simulink library "PC_Simulator_Lib"  (Simulink 8.2)
settings: Solver=ode45  StartTime=0.0  StopTime=10.0  RelTol=1e-3
values from neighbouring files (symbols this model uses):
  data = [r1 r2 r3 r4 L1 L2 L3 L4]    [strasse_Bedatung_HNI_ITI.m]
  distSameLane = 60    [InitialisationsEnv.m]
  eng_speed = [0 60 120 180 240 300 360 420 480 540 600 660 ... (101 elements, 1x101)]    [engine_table.mat]    (also in motor_parameter_calc.m = omega)
  Heading_init = 0    [Start.m]
  inertiaLateral = 25*(radiusWheel)^2    (= 4.129024)    [Start.m]
  laneWidth = 3.6    [InitialisationsEnv.m]    (also in strasse_Bedatung_HNI_ITI.m)
  omega_engine = [0.000000 150.000000 500.000000 1000.000000 1500.000000 2000.000000 2500.000000 3000.000000 3500.000000 4000.000000 4500.000000 5000.000000 5500.000000 6000.000000]    [friction_tables.m]
  omega_max = 6000    [engine_table.mat]    (also in motor_parameter_calc.m)
  omega_wheel = [0 20 40 60 80 100 122 143.7 164]    [friction_tables.m]
  para_Fellow_8_Points = ADAS.Fellow_8_Points    [ADAS_parameters.m]
  position_start_x = [x1 x2 x3 x4 x5 x6 x7]    [strasse_Bedatung_HNI_ITI.m]
  position_start_y = [y1 y2 y3 y4 y5 y6 y7]    [strasse_Bedatung_HNI_ITI.m]
  rad3rdLine = 57.2    [InitialisationsEnv.m]    (also in strasse_Bedatung_HNI_ITI.m)
  radiusWheel = 16*2.54/100    (= 0.4064)    [Start.m]
  s_values = [S1 S2 S3 S4 S5 S6 S7]    [strasse_Bedatung_HNI_ITI.m]
  segmentLimits = [segment1EndThirdLine                   segment2EndThirdLine                   segment3EndThirdLine                   segment4EndThirdLine                   segment5EndThirdLine                   segment6EndThirdLine                   segment7EndThirdLine                   segment8EndThirdLine                   ]    [InitialisationsEnv.m]    (also in strasse_Bedatung_HNI_ITI.m)
  setPosT = [-1.8 -5.4 -1.8 -5.4 -1.8 -5.4 -1.8 -5.4 -1.8 -5.4]    [InitialisationsEnv.m]
  torque = [297.089227105 300.997600937 304.800343044 308.497453426 312.088932082 315.574779014 318.95499422 322.229577701 325.398529457 328.461849487 331.419537793 334.271594373 ... (101 elements, 1x101)]    [engine_table.mat]    (also in motor_parameter_calc.m = g)
  Torque_lost = [0.000000 -8.777780 -15.000000 -26.800000 -29.600000 -32.700000 -35.900000 -39.300000 -42.800000 -46.500000 -50.300000 -54.300000 -58.500000 -62.800000 ]*0.6    [friction_tables.m]
  Torque_lost_wheel = [0.8 0.8 0.75 0.7 0.4 0.3 0.2 0.07 0.07]*0.2    [friction_tables.m]
  X_init = 0    [Start.m]
  Y_init = 1.8    [Start.m]
  Z_init = 0    [Start.m]
undefined symbols (not defined in the file or in its folder): Acc_Pedal, ADAS, Brake_Pedal, Joystick, Newton, Para, Raphson, Standard_Devices, Steering_Wheel_Angle, UDP_Protocol
libraries: simulink x43, rtwinlib x7, dspnetwork x2, simulink_extras x1, vrlib x1
(part 3 of 13)

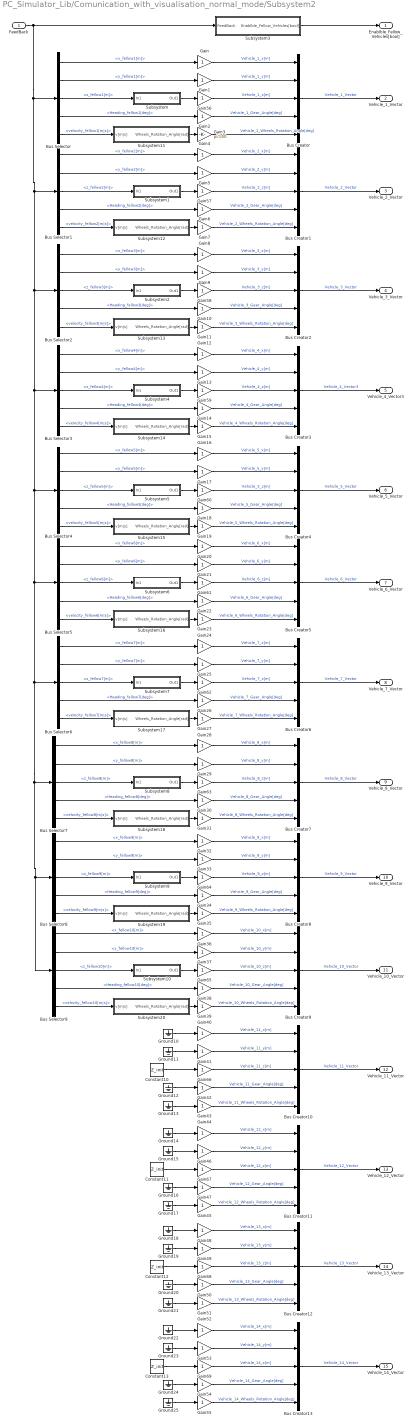
== system PC_Simulator_Lib/Comunication_with_visualisation_normal_mode/Subsystem2 ==
  FeedBack : Inport
  Bus Creator{,1..13} (14 alike) : BusCreator  Inputs=5
  Bus Selector : BusSelector  OutputSignals=Environment.fellow_car_1.x_fellow1[m],Environment.fellow_car_1.y_fellow1[m],Environment.fellow_car_1.z_fellow1[m],Environment.fellow_car_1.Heading_fellow1[deg],Environment.fellow_car_1.velocity_fellow1[m|s]
  Bus Selector1 : BusSelector  OutputSignals=Environment.fellow_car_2.x_fellow2[m],Environment.fellow_car_2.y_fellow2[m],Environment.fellow_car_2.z_fellow2[m],Environment.fellow_car_2.Heading_fellow2[deg],Environment.fellow_car_2.velocity_fellow2[m|s]
  Bus Selector2 : BusSelector  OutputSignals=Environment.fellow_car_3.x_fellow3[m],Environment.fellow_car_3.y_fellow3[m],Environment.fellow_car_3.z_fellow3[m],Environment.fellow_car_3.Heading_fellow3[deg],Environment.fellow_car_3.velocity_fellow3[m|s]
  Bus Selector3 : BusSelector  OutputSignals=Environment.fellow_car_4.x_fellow4[m],Environment.fellow_car_4.y_fellow4[m],Environment.fellow_car_4.z_fellow4[m],Environment.fellow_car_4.Heading_fellow4[deg],Environment.fellow_car_4.velocity_fellow4[m|s]
  Bus Selector4 : BusSelector  OutputSignals=Environment.fellow_car_5.x_fellow5[m],Environment.fellow_car_5.y_fellow5[m],Environment.fellow_car_5.z_fellow5[m],Environment.fellow_car_5.Heading_fellow5[deg],Environment.fellow_car_5.velocity_fellow5[m|s]
  Bus Selector5 : BusSelector  OutputSignals=Environment.fellow_car_6.x_fellow6[m],Environment.fellow_car_6.y_fellow6[m],Environment.fellow_car_6.z_fellow6[m],Environment.fellow_car_6.Heading_fellow6[deg],Environment.fellow_car_6.velocity_fellow6[m|s]
  Bus Selector6 : BusSelector  OutputSignals=Environment.fellow_car_7.x_fellow7[m],Environment.fellow_car_7.y_fellow7[m],Environment.fellow_car_7.z_fellow7[m],Environment.fellow_car_7.Heading_fellow7[deg],Environment.fellow_car_7.velocity_fellow7[m|s]
  Bus Selector7 : BusSelector  OutputSignals=Environment.fellow_car_8.x_fellow8[m],Environment.fellow_car_8.y_fellow8[m],Environment.fellow_car_8.z_fellow8[m],Environment.fellow_car_8.Heading_fellow8[deg],Environment.fellow_car_8.velocity_fellow8[m|s]
  Bus Selector8 : BusSelector  OutputSignals=Environment.fellow_car_9.x_fellow9[m],Environment.fellow_car_9.y_fellow9[m],Environment.fellow_car_9.z_fellow9[m],Environment.fellow_car_9.Heading_fellow9[deg],Environment.fellow_car_9.velocity_fellow9[m|s]
  Bus Selector9 : BusSelector  OutputSignals=Environment.fellow_car_10.x_fellow10[m],Environment.fellow_car_10.y_fellow10[m],Environment.fellow_car_10.z_fellow10[m],Environment.fellow_car_10.Heading_fellow10[deg],Environment.fellow_car_10.velocity_fellow10[m|s]
  Constant{10..13} (4 alike) : Constant  Value=Z_init
  Gain{,1..2,4..69} (69 alike) : Gain
  Gain3 : Gain  Gain=pi/180
  Ground{10..25} (16 alike) : Ground
  Subsystem : Subsystem
  Subsystem1 : Subsystem
  Subsystem10 : Subsystem
  Subsystem11 : Subsystem
  Subsystem12 : Subsystem
  Subsystem13 : Subsystem
  Subsystem14 : Subsystem
  Subsystem15 : Subsystem
  Subsystem16 : Subsystem
  Subsystem17 : Subsystem
  Subsystem18 : Subsystem
  Subsystem19 : Subsystem
  Subsystem2 : Subsystem
  Subsystem20 : Subsystem
  Subsystem3 : Subsystem
  Subsystem4 : Subsystem
  Subsystem5 : Subsystem
  Subsystem6 : Subsystem
  Subsystem7 : Subsystem
  Subsystem8 : Subsystem
  Subsystem9 : Subsystem
  Enablble_Fellow_Vehicles[bool] : Outport
  Vehicle_1_Vector : Outport  Port=2
  Vehicle_2_Vector : Outport  Port=3
  Vehicle_3_Vector : Outport  Port=4
  Vehicle_4_Vector3 : Outport  Port=5
  Vehicle_5_Vector : Outport  Port=6
  Vehicle_6_Vector : Outport  Port=7
  Vehicle_7_Vector : Outport  Port=8
  Vehicle_8_Vector : Outport  Port=9
  Vehicle_9_Vector : Outport  Port=10
  Vehicle_10_Vector : Outport  Port=11
  Vehicle_11_Vector : Outport  Port=12
  Vehicle_12_Vector : Outport  Port=13
  Vehicle_13_Vector : Outport  Port=14
  Vehicle_14_Vector : Outport  Port=15
  wires:
  Bus Creator/1 -> Vehicle_1_Vector/1  "Vehicle_1_Vector"
  Bus Creator1/1 -> Vehicle_2_Vector/1  "Vehicle_2_Vector"
  Bus Creator2/1 -> Vehicle_3_Vector/1  "Vehicle_3_Vector"
  Bus Creator3/1 -> Vehicle_4_Vector3/1  "Vehicle_4_Vector3"
  Bus Creator4/1 -> Vehicle_5_Vector/1  "Vehicle_5_Vector"
  Bus Creator5/1 -> Vehicle_6_Vector/1  "Vehicle_6_Vector"
  Bus Creator6/1 -> Vehicle_7_Vector/1  "Vehicle_7_Vector"
  Bus Creator7/1 -> Vehicle_8_Vector/1  "Vehicle_8_Vector"
  Bus Creator8/1 -> Vehicle_9_Vector/1  "Vehicle_9_Vector"
  Bus Creator9/1 -> Vehicle_10_Vector/1  "Vehicle_10_Vector"
  Bus Creator10/1 -> Vehicle_11_Vector/1  "Vehicle_11_Vector"
  Bus Creator11/1 -> Vehicle_12_Vector/1  "Vehicle_12_Vector"
  Bus Creator12/1 -> Vehicle_13_Vector/1  "Vehicle_13_Vector"
  Bus Creator13/1 -> Vehicle_14_Vector/1  "Vehicle_14_Vector"
  Gain/1 -> Bus Creator/1  "Vehicle_1_x[m]"
  Gain1/1 -> Bus Creator/2  "Vehicle_1_y[m]"
  Gain56/1 -> Bus Creator/3  "Vehicle_1_z[m]"
  Gain2/1 -> Bus Creator/4  "Vehicle_1_Gear_Angle[deg]"
  Gain3/1 -> Bus Creator/5  "Vehicle_1_Wheels_Rotation_Angle[deg]"
  Gain4/1 -> Bus Creator1/1  "Vehicle_2_x[m]"
  Gain5/1 -> Bus Creator1/2  "Vehicle_2_y[m]"
  Gain57/1 -> Bus Creator1/3  "Vehicle_2_z[m]"
  Gain6/1 -> Bus Creator1/4  "Vehicle_2_Gear_Angle[deg]"
  Gain7/1 -> Bus Creator1/5  "Vehicle_2_Wheels_Rotation_Angle[deg]"
  Gain8/1 -> Bus Creator2/1  "Vehicle_3_x[m]"
  Gain9/1 -> Bus Creator2/2  "Vehicle_3_y[m]"
  Gain58/1 -> Bus Creator2/3  "Vehicle_3_z[m]"
  Gain10/1 -> Bus Creator2/4  "Vehicle_3_Gear_Angle[deg]"
  Gain11/1 -> Bus Creator2/5  "Vehicle_3_Wheels_Rotation_Angle[deg]"
  Gain12/1 -> Bus Creator3/1  "Vehicle_4_x[m]"
  Gain13/1 -> Bus Creator3/2  "Vehicle_4_y[m]"
  Gain59/1 -> Bus Creator3/3  "Vehicle_4_z[m]"
  Gain14/1 -> Bus Creator3/4  "Vehicle_4_Gear_Angle[deg]"
  Gain15/1 -> Bus Creator3/5  "Vehicle_4_Wheels_Rotation_Angle[deg]"
  Gain16/1 -> Bus Creator4/1  "Vehicle_5_x[m]"
  Gain17/1 -> Bus Creator4/2  "Vehicle_5_y[m]"
  Gain60/1 -> Bus Creator4/3  "Vehicle_5_z[m]"
  Gain18/1 -> Bus Creator4/4  "Vehicle_5_Gear_Angle[deg]"
  Gain19/1 -> Bus Creator4/5  "Vehicle_5_Wheels_Rotation_Angle[deg]"
  Gain20/1 -> Bus Creator5/1  "Vehicle_6_x[m]"
  Gain21/1 -> Bus Creator5/2  "Vehicle_6_y[m]"
  Gain61/1 -> Bus Creator5/3  "Vehicle_6_z[m]"
  Gain22/1 -> Bus Creator5/4  "Vehicle_6_Gear_Angle[deg]"
  Gain23/1 -> Bus Creator5/5  "Vehicle_6_Wheels_Rotation_Angle[deg]"
  Gain24/1 -> Bus Creator6/1  "Vehicle_7_x[m]"
  Gain25/1 -> Bus Creator6/2  "Vehicle_7_y[m]"
  Gain62/1 -> Bus Creator6/3  "Vehicle_7_z[m]"
  Gain26/1 -> Bus Creator6/4  "Vehicle_7_Gear_Angle[deg]"
  Gain27/1 -> Bus Creator6/5  "Vehicle_7_Wheels_Rotation_Angle[deg]"
  Gain28/1 -> Bus Creator7/1  "Vehicle_8_x[m]"
  Gain29/1 -> Bus Creator7/2  "Vehicle_8_y[m]"
  Gain63/1 -> Bus Creator7/3  "Vehicle_8_z[m]"
  Gain30/1 -> Bus Creator7/4  "Vehicle_8_Gear_Angle[deg]"
  Gain31/1 -> Bus Creator7/5  "Vehicle_8_Wheels_Rotation_Angle[deg]"
  Gain32/1 -> Bus Creator8/1  "Vehicle_9_x[m]"
  Gain33/1 -> Bus Creator8/2  "Vehicle_9_y[m]"
  Gain64/1 -> Bus Creator8/3  "Vehicle_9_z[m]"
  Gain34/1 -> Bus Creator8/4  "Vehicle_9_Gear_Angle[deg]"
  Gain35/1 -> Bus Creator8/5  "Vehicle_9_Wheels_Rotation_Angle[deg]"
  Gain36/1 -> Bus Creator9/1  "Vehicle_10_x[m]"
  Gain37/1 -> Bus Creator9/2  "Vehicle_10_y[m]"
  Gain65/1 -> Bus Creator9/3  "Vehicle_10_z[m]"
  Gain38/1 -> Bus Creator9/4  "Vehicle_10_Gear_Angle[deg]"
  Gain39/1 -> Bus Creator9/5  "Vehicle_10_Wheels_Rotation_Angle[deg]"
  Gain40/1 -> Bus Creator10/1  "Vehicle_11_x[m]"
  Gain41/1 -> Bus Creator10/2  "Vehicle_11_y[m]"
  Gain66/1 -> Bus Creator10/3  "Vehicle_11_z[m]"
  Gain42/1 -> Bus Creator10/4  "Vehicle_11_Gear_Angle[deg]"
  Gain43/1 -> Bus Creator10/5  "Vehicle_11_Wheels_Rotation_Angle[deg]"
  Gain44/1 -> Bus Creator11/1  "Vehicle_12_x[m]"
  Gain46/1 -> Bus Creator11/2  "Vehicle_12_y[m]"
  Gain67/1 -> Bus Creator11/3  "Vehicle_12_z[m]"
  Gain47/1 -> Bus Creator11/4  "Vehicle_12_Gear_Angle[deg]"
  Gain45/1 -> Bus Creator11/5  "Vehicle_12_Wheels_Rotation_Angle[deg]"
  Gain48/1 -> Bus Creator12/1  "Vehicle_13_x[m]"
  Gain49/1 -> Bus Creator12/2  "Vehicle_13_y[m]"
  Gain68/1 -> Bus Creator12/3  "Vehicle_13_z[m]"
  Gain50/1 -> Bus Creator12/4  "Vehicle_13_Gear_Angle[deg]"
  Gain51/1 -> Bus Creator12/5  "Vehicle_13_Wheels_Rotation_Angle[deg]"
  Gain52/1 -> Bus Creator13/1  "Vehicle_14_x[m]"
  Gain53/1 -> Bus Creator13/2  "Vehicle_14_y[m]"
  Gain69/1 -> Bus Creator13/3  "Vehicle_14_z[m]"
  Gain54/1 -> Bus Creator13/4  "Vehicle_14_Gear_Angle[deg]"
  Gain55/1 -> Bus Creator13/5  "Vehicle_14_Wheels_Rotation_Angle[deg]"
  Subsystem3/1(Enablble_Fellow_Vehicles[bool]) -> Enablble_Fellow_Vehicles[bool]/1
  Subsystem5/1(Out1) -> Gain60/1
  Subsystem6/1(Out1) -> Gain61/1
  Subsystem7/1(Out1) -> Gain62/1
  Subsystem8/1(Out1) -> Gain63/1
  Subsystem9/1(Out1) -> Gain64/1
  Subsystem10/1(Out1) -> Gain65/1
  Constant10/1 -> Gain66/1
  Constant11/1 -> Gain67/1
  Constant12/1 -> Gain68/1
  Constant13/1 -> Gain69/1
  Subsystem/1(Out1) -> Gain56/1
  Bus Selector/1 -> Gain/1  "<x_fellow1[m]>"
  Bus Selector/2 -> Gain1/1  "<y_fellow1[m]>"
  Bus Selector/3 -> Subsystem/1(In1)  "<z_fellow1[m]>"
  Bus Selector/4 -> Gain2/1  "<Heading_fellow1[deg]>"
  Ground10/1 -> Gain40/1
  Ground11/1 -> Gain41/1
  Ground12/1 -> Gain42/1
  Ground13/1 -> Gain43/1
  Ground14/1 -> Gain44/1
  Ground15/1 -> Gain46/1
  Ground16/1 -> Gain47/1
  Ground17/1 -> Gain45/1
  Ground18/1 -> Gain48/1
  Ground19/1 -> Gain49/1
  Ground20/1 -> Gain50/1
  Ground21/1 -> Gain51/1
  Ground22/1 -> Gain52/1
  Ground23/1 -> Gain53/1
  Ground24/1 -> Gain54/1
  Ground25/1 -> Gain55/1
  Subsystem1/1(Out1) -> Gain57/1
  Subsystem2/1(Out1) -> Gain58/1
  Subsystem4/1(Out1) -> Gain59/1
  FeedBack/1 -> Bus Selector9/1, Bus Selector8/1, Bus Selector7/1, Bus Selector6/1, Bus Selector5/1, Bus Selector4/1, Bus Selector3/1, Bus Selector2/1, Bus Selector1/1, Bus Selector/1, Subsystem3/1(FeedBack)
  Bus Selector1/3 -> Subsystem1/1(In1)  "<z_fellow2[m]>"
  Bus Selector1/1 -> Gain4/1  "<x_fellow2[m]>"
  Bus Selector1/2 -> Gain5/1  "<y_fellow2[m]>"
  Bus Selector1/4 -> Gain6/1  "<Heading_fellow2[deg]>"
  Bus Selector2/3 -> Subsystem2/1(In1)  "<z_fellow3[m]>"
  Bus Selector2/1 -> Gain8/1  "<x_fellow3[m]>"
  Bus Selector2/2 -> Gain9/1  "<y_fellow3[m]>"
  Bus Selector2/4 -> Gain10/1  "<Heading_fellow3[deg]>"
  Bus Selector3/3 -> Subsystem4/1(In1)  "<z_fellow4[m]>"
  Bus Selector3/1 -> Gain12/1  "<x_fellow4[m]>"
  Bus Selector3/2 -> Gain13/1  "<y_fellow4[m]>"
  Bus Selector3/4 -> Gain14/1  "<Heading_fellow4[deg]>"
  Bus Selector4/3 -> Subsystem5/1(In1)  "<z_fellow5[m]>"
  Bus Selector4/1 -> Gain16/1  "<x_fellow5[m]>"
  Bus Selector4/2 -> Gain17/1  "<y_fellow5[m]>"
  Bus Selector4/4 -> Gain18/1  "<Heading_fellow5[deg]>"
  Bus Selector5/3 -> Subsystem6/1(In1)  "<z_fellow6[m]>"
  Bus Selector5/1 -> Gain20/1  "<x_fellow6[m]>"
  Bus Selector5/2 -> Gain21/1  "<y_fellow6[m]>"
  Bus Selector5/4 -> Gain22/1  "<Heading_fellow6[deg]>"
  Bus Selector6/3 -> Subsystem7/1(In1)  "<z_fellow7[m]>"
  Bus Selector6/1 -> Gain24/1  "<x_fellow7[m]>"
  Bus Selector6/2 -> Gain25/1  "<y_fellow7[m]>"
  Bus Selector6/4 -> Gain26/1  "<Heading_fellow7[deg]>"
  Bus Selector7/3 -> Subsystem8/1(In1)  "<z_fellow8[m]>"
  Bus Selector7/1 -> Gain28/1  "<x_fellow8[m]>"
  Bus Selector7/2 -> Gain29/1  "<y_fellow8[m]>"
  Bus Selector7/4 -> Gain30/1  "<Heading_fellow8[deg]>"
  Bus Selector8/3 -> Subsystem9/1(In1)  "<z_fellow9[m]>"
  Bus Selector8/1 -> Gain32/1  "<x_fellow9[m]>"
  Bus Selector8/2 -> Gain33/1  "<y_fellow9[m]>"
  Bus Selector8/4 -> Gain34/1  "<Heading_fellow9[deg]>"
  Bus Selector9/3 -> Subsystem10/1(In1)  "<z_fellow10[m]>"
  Bus Selector9/1 -> Gain36/1  "<x_fellow10[m]>"
  Bus Selector9/2 -> Gain37/1  "<y_fellow10[m]>"
  Bus Selector9/4 -> Gain38/1  "<Heading_fellow10[deg]>"
  Subsystem11/1(Wheels_Rotation_Angle[rad]) -> Gain3/1
  Subsystem12/1(Wheels_Rotation_Angle[rad]) -> Gain7/1
  Subsystem13/1(Wheels_Rotation_Angle[rad]) -> Gain11/1
  Subsystem14/1(Wheels_Rotation_Angle[rad]) -> Gain15/1
  Subsystem15/1(Wheels_Rotation_Angle[rad]) -> Gain19/1
  Subsystem16/1(Wheels_Rotation_Angle[rad]) -> Gain23/1
  Subsystem17/1(Wheels_Rotation_Angle[rad]) -> Gain27/1
  Subsystem18/1(Wheels_Rotation_Angle[rad]) -> Gain31/1
  Subsystem19/1(Wheels_Rotation_Angle[rad]) -> Gain35/1
  Subsystem20/1(Wheels_Rotation_Angle[rad]) -> Gain39/1
  Bus Selector/5 -> Subsystem11/1(v[m|s])  "<velocity_fellow1[m|s]>"
  Bus Selector1/5 -> Subsystem12/1(v[m|s])  "<velocity_fellow2[m|s]>"
  Bus Selector9/5 -> Subsystem20/1(v[m|s])  "<velocity_fellow10[m|s]>"
  Bus Selector8/5 -> Subsystem19/1(v[m|s])  "<velocity_fellow9[m|s]>"
  Bus Selector7/5 -> Subsystem18/1(v[m|s])  "<velocity_fellow8[m|s]>"
  Bus Selector6/5 -> Subsystem17/1(v[m|s])  "<velocity_fellow7[m|s]>"
  Bus Selector5/5 -> Subsystem16/1(v[m|s])  "<velocity_fellow6[m|s]>"
  Bus Selector4/5 -> Subsystem15/1(v[m|s])  "<velocity_fellow5[m|s]>"
  Bus Selector3/5 -> Subsystem14/1(v[m|s])  "<velocity_fellow4[m|s]>"
  Bus Selector2/5 -> Subsystem13/1(v[m|s])  "<velocity_fellow3[m|s]>"

== system PC_Simulator_Lib/Comunication_with_visualisation_normal_mode/Subsystem3 ==
  In1 : Inport
  Add : Sum
  Constant : Constant  Value=1000
  Gain1 : Gain  Gain=60/(2*pi)
  Out1 : Outport
  wires:
  In1/1 -> Gain1/1
  Add/1 -> Out1/1
  Gain1/1 -> Add/1
  Constant/1 -> Add/2

== system PC_Simulator_Lib/Comunication_with_visualisation_normal_mode/Subsystem4 ==
  In1 : Inport
  Gain : Gain  Gain=1/radiusWheel
  Integrator : Integrator
  Out1 : Outport
  wires:
  Integrator/1 -> Out1/1
  In1/1 -> Gain/1
  Gain/1 -> Integrator/1

== system PC_Simulator_Lib/Comunication_with_visualisation_normal_mode/Subsystem5 ==
  In1 : Inport
  Add : Sum
  Bus Selector3 : BusSelector  OutputSignals=Vehicle_Dynamics.Wheel_Steering_Angle_Left[rad],Vehicle_Dynamics.Wheel_Steering_Angle_Right[rad]
  Gain : Gain  Gain=-0.5
  Gain1 : Gain  Gain=180/pi
  Out1 : Outport
  wires:
  In1/1 -> Bus Selector3/1
  Bus Selector3/1 -> Add/1  "<Wheel_Steering_Angle_Left[rad]>"
  Bus Selector3/2 -> Add/2  "<Wheel_Steering_Angle_Right[rad]>"
  Add/1 -> Gain/1
  Gain/1 -> Gain1/1
  Gain1/1 -> Out1/1

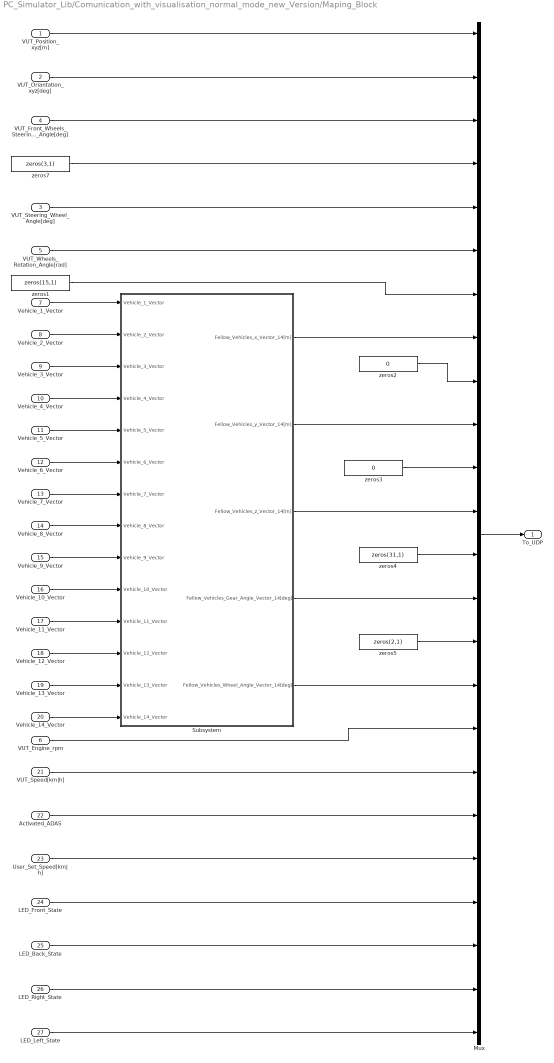
== system PC_Simulator_Lib/Comunication_with_visualisation_normal_mode_new_Version/Maping_Block ==
  VUT_Position_xyz[m] : Inport
  VUT_Oriantation_xyz[deg] : Inport  Port=2
  VUT_Steering_Wheel_Angle[deg] : Inport  Port=3
  VUT_Front_Wheels_Steering_Angle[deg] : Inport  Port=4
  VUT_Wheels_Rotation_Angle[rad] : Inport  Port=5
  VUT_Engine_rpm : Inport  Port=6
  Vehicle_1_Vector : Inport  Port=7
  Vehicle_2_Vector : Inport  Port=8
  Vehicle_3_Vector : Inport  Port=9
  Vehicle_4_Vector : Inport  Port=10
  Vehicle_5_Vector : Inport  Port=11
  Vehicle_6_Vector : Inport  Port=12
  Vehicle_7_Vector : Inport  Port=13
  Vehicle_8_Vector : Inport  Port=14
  Vehicle_9_Vector : Inport  Port=15
  Vehicle_10_Vector : Inport  Port=16
  Vehicle_11_Vector : Inport  Port=17
  Vehicle_12_Vector : Inport  Port=18
  Vehicle_13_Vector : Inport  Port=19
  Vehicle_14_Vector : Inport  Port=20
  VUT_Speed[km|h] : Inport  Port=21
  Activated_ADAS : Inport  Port=22
  User_Set_Speed[km|h] : Inport  Port=23
  LED_Front_State : Inport  Port=24
  LED_Back_State : Inport  Port=25
  LED_Right_State : Inport  Port=26
  LED_Left_State : Inport  Port=27
  Mux : Mux  Inputs=24
  Subsystem : Subsystem
  zeros1 : Constant  Value=zeros(15,1)
  zeros2 : Constant  Value=0
  zeros3 : Constant  Value=0
  zeros4 : Constant  Value=zeros(31,1)
  zeros5 : Constant  Value=zeros(2,1)
  zeros7 : Constant  Value=zeros(3,1)
  To_UDP : Outport
  wires:
  LED_Back_State/1 -> Mux/22
  LED_Right_State/1 -> Mux/23
  LED_Left_State/1 -> Mux/24
  LED_Front_State/1 -> Mux/21
  User_Set_Speed[km|h]/1 -> Mux/20
  VUT_Speed[km|h]/1 -> Mux/18
  Activated_ADAS/1 -> Mux/19
  Mux/1 -> To_UDP/1
  VUT_Engine_rpm/1 -> Mux/17
  Subsystem/5(Fellow_Vehicles_Wheel_Angle_Vector_14[deg]) -> Mux/16
  zeros5/1 -> Mux/15
  Subsystem/4(Fellow_Vehicles_Gear_Angle_Vector_14[deg]) -> Mux/14
  zeros4/1 -> Mux/13
  Subsystem/3(Fellow_Vehicles_z_Vector_14[m]) -> Mux/12
  zeros3/1 -> Mux/11
  Subsystem/2(Fellow_Vehicles_y_Vector_14[m]) -> Mux/10
  zeros2/1 -> Mux/9
  Subsystem/1(Fellow_Vehicles_x_Vector_14[m]) -> Mux/8
  Vehicle_8_Vector/1 -> Subsystem/8(Vehicle_8_Vector)
  Vehicle_11_Vector/1 -> Subsystem/11(Vehicle_11_Vector)
  Vehicle_10_Vector/1 -> Subsystem/10(Vehicle_10_Vector)
  Vehicle_9_Vector/1 -> Subsystem/9(Vehicle_9_Vector)
  Vehicle_12_Vector/1 -> Subsystem/12(Vehicle_12_Vector)
  Vehicle_13_Vector/1 -> Subsystem/13(Vehicle_13_Vector)
  Vehicle_14_Vector/1 -> Subsystem/14(Vehicle_14_Vector)
  Vehicle_1_Vector/1 -> Subsystem/1(Vehicle_1_Vector)
  Vehicle_2_Vector/1 -> Subsystem/2(Vehicle_2_Vector)
  Vehicle_3_Vector/1 -> Subsystem/3(Vehicle_3_Vector)
  Vehicle_4_Vector/1 -> Subsystem/4(Vehicle_4_Vector)
  Vehicle_5_Vector/1 -> Subsystem/5(Vehicle_5_Vector)
  Vehicle_6_Vector/1 -> Subsystem/6(Vehicle_6_Vector)
  Vehicle_7_Vector/1 -> Subsystem/7(Vehicle_7_Vector)
  zeros1/1 -> Mux/7
  VUT_Wheels_Rotation_Angle[rad]/1 -> Mux/6
  VUT_Front_Wheels_Steering_Angle[deg]/1 -> Mux/3
  zeros7/1 -> Mux/4
  VUT_Steering_Wheel_Angle[deg]/1 -> Mux/5
  VUT_Oriantation_xyz[deg]/1 -> Mux/2
  VUT_Position_xyz[m]/1 -> Mux/1

== system PC_Simulator_Lib/Comunication_with_visualisation_normal_mode_new_Version/Subsystem ==
  In1 : Inport
  Bus Selector : BusSelector  OutputSignals=x_CoG[m],y_CoG[m],z_CoG[m]
  Mux : Mux  Inputs=3
  Out1 : Outport
  wires:
  Bus Selector/1 -> Mux/1  "<x_CoG[m]>"
  Bus Selector/2 -> Mux/2  "<y_CoG[m]>"
  Bus Selector/3 -> Mux/3  "<z_CoG[m]>"
  Mux/1 -> Out1/1
  In1/1 -> Bus Selector/1

== system PC_Simulator_Lib/Comunication_with_visualisation_normal_mode_new_Version/Subsystem1 ==
  In1 : Inport
  Bus Selector : BusSelector  OutputSignals=Pitch_Angle,Roll_Angle,Yaw_Angle
  Mux : Mux  Inputs=3
  Out1 : Outport
  wires:
  In1/1 -> Bus Selector/1
  Mux/1 -> Out1/1
  Bus Selector/3 -> Mux/3  "<Yaw_Angle>"
  Bus Selector/2 -> Mux/2  "<Roll_Angle>"
  Bus Selector/1 -> Mux/1  "<Pitch_Angle>"

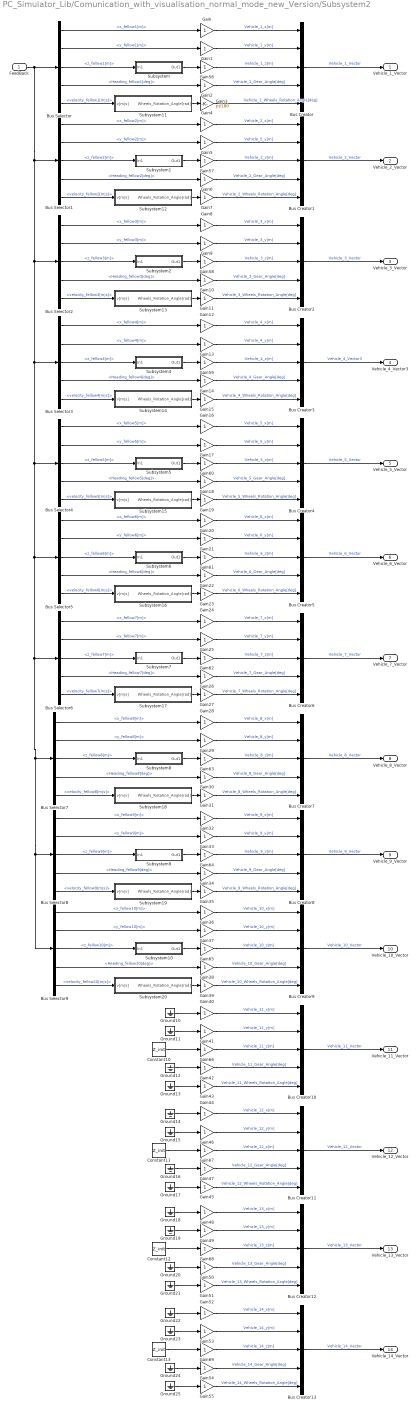
== system PC_Simulator_Lib/Comunication_with_visualisation_normal_mode_new_Version/Subsystem2 ==
  FeedBack : Inport
  Bus Creator{,1..13} (14 alike) : BusCreator  Inputs=5
  Bus Selector : BusSelector  OutputSignals=Environment.fellow_car_1.x_fellow1[m],Environment.fellow_car_1.y_fellow1[m],Environment.fellow_car_1.z_fellow1[m],Environment.fellow_car_1.Heading_fellow1[deg],Environment.fellow_car_1.velocity_fellow1[m|s]
  Bus Selector1 : BusSelector  OutputSignals=Environment.fellow_car_2.x_fellow2[m],Environment.fellow_car_2.y_fellow2[m],Environment.fellow_car_2.z_fellow2[m],Environment.fellow_car_2.Heading_fellow2[deg],Environment.fellow_car_2.velocity_fellow2[m|s]
  Bus Selector2 : BusSelector  OutputSignals=Environment.fellow_car_3.x_fellow3[m],Environment.fellow_car_3.y_fellow3[m],Environment.fellow_car_3.z_fellow3[m],Environment.fellow_car_3.Heading_fellow3[deg],Environment.fellow_car_3.velocity_fellow3[m|s]
  Bus Selector3 : BusSelector  OutputSignals=Environment.fellow_car_4.x_fellow4[m],Environment.fellow_car_4.y_fellow4[m],Environment.fellow_car_4.z_fellow4[m],Environment.fellow_car_4.Heading_fellow4[deg],Environment.fellow_car_4.velocity_fellow4[m|s]
  Bus Selector4 : BusSelector  OutputSignals=Environment.fellow_car_5.x_fellow5[m],Environment.fellow_car_5.y_fellow5[m],Environment.fellow_car_5.z_fellow5[m],Environment.fellow_car_5.Heading_fellow5[deg],Environment.fellow_car_5.velocity_fellow5[m|s]
  Bus Selector5 : BusSelector  OutputSignals=Environment.fellow_car_6.x_fellow6[m],Environment.fellow_car_6.y_fellow6[m],Environment.fellow_car_6.z_fellow6[m],Environment.fellow_car_6.Heading_fellow6[deg],Environment.fellow_car_6.velocity_fellow6[m|s]
  Bus Selector6 : BusSelector  OutputSignals=Environment.fellow_car_7.x_fellow7[m],Environment.fellow_car_7.y_fellow7[m],Environment.fellow_car_7.z_fellow7[m],Environment.fellow_car_7.Heading_fellow7[deg],Environment.fellow_car_7.velocity_fellow7[m|s]
  Bus Selector7 : BusSelector  OutputSignals=Environment.fellow_car_8.x_fellow8[m],Environment.fellow_car_8.y_fellow8[m],Environment.fellow_car_8.z_fellow8[m],Environment.fellow_car_8.Heading_fellow8[deg],Environment.fellow_car_8.velocity_fellow8[m|s]
  Bus Selector8 : BusSelector  OutputSignals=Environment.fellow_car_9.x_fellow9[m],Environment.fellow_car_9.y_fellow9[m],Environment.fellow_car_9.z_fellow9[m],Environment.fellow_car_9.Heading_fellow9[deg],Environment.fellow_car_9.velocity_fellow9[m|s]
  Bus Selector9 : BusSelector  OutputSignals=Environment.fellow_car_10.x_fellow10[m],Environment.fellow_car_10.y_fellow10[m],Environment.fellow_car_10.z_fellow10[m],Environment.fellow_car_10.Heading_fellow10[deg],Environment.fellow_car_10.velocity_fellow10[m|s]
  Constant{10..13} (4 alike) : Constant  Value=Z_init
  Gain{,1..2,4..69} (69 alike) : Gain
  Gain3 : Gain  Gain=pi/180
  Ground{10..25} (16 alike) : Ground
  Subsystem : Subsystem
  Subsystem1 : Subsystem
  Subsystem10 : Subsystem
  Subsystem11 : Subsystem
  Subsystem12 : Subsystem
  Subsystem13 : Subsystem
  Subsystem14 : Subsystem
  Subsystem15 : Subsystem
  Subsystem16 : Subsystem
  Subsystem17 : Subsystem
  Subsystem18 : Subsystem
  Subsystem19 : Subsystem
  Subsystem2 : Subsystem
  Subsystem20 : Subsystem
  Subsystem4 : Subsystem
  Subsystem5 : Subsystem
  Subsystem6 : Subsystem
  Subsystem7 : Subsystem
  Subsystem8 : Subsystem
  Subsystem9 : Subsystem
  Vehicle_1_Vector : Outport
  Vehicle_2_Vector : Outport  Port=2
  Vehicle_3_Vector : Outport  Port=3
  Vehicle_4_Vector3 : Outport  Port=4
  Vehicle_5_Vector : Outport  Port=5
  Vehicle_6_Vector : Outport  Port=6
  Vehicle_7_Vector : Outport  Port=7
  Vehicle_8_Vector : Outport  Port=8
  Vehicle_9_Vector : Outport  Port=9
  Vehicle_10_Vector : Outport  Port=10
  Vehicle_11_Vector : Outport  Port=11
  Vehicle_12_Vector : Outport  Port=12
  Vehicle_13_Vector : Outport  Port=13
  Vehicle_14_Vector : Outport  Port=14
  wires:
  Bus Selector2/5 -> Subsystem13/1(v[m|s])  "<velocity_fellow3[m|s]>"
  Bus Selector3/5 -> Subsystem14/1(v[m|s])  "<velocity_fellow4[m|s]>"
  Bus Selector4/5 -> Subsystem15/1(v[m|s])  "<velocity_fellow5[m|s]>"
  Bus Selector5/5 -> Subsystem16/1(v[m|s])  "<velocity_fellow6[m|s]>"
  Bus Selector6/5 -> Subsystem17/1(v[m|s])  "<velocity_fellow7[m|s]>"
  Bus Selector7/5 -> Subsystem18/1(v[m|s])  "<velocity_fellow8[m|s]>"
  Bus Selector8/5 -> Subsystem19/1(v[m|s])  "<velocity_fellow9[m|s]>"
  Bus Selector9/5 -> Subsystem20/1(v[m|s])  "<velocity_fellow10[m|s]>"
  Bus Selector1/5 -> Subsystem12/1(v[m|s])  "<velocity_fellow2[m|s]>"
  Bus Selector/5 -> Subsystem11/1(v[m|s])  "<velocity_fellow1[m|s]>"
  Subsystem20/1(Wheels_Rotation_Angle[rad]) -> Gain39/1
  Subsystem19/1(Wheels_Rotation_Angle[rad]) -> Gain35/1
  Subsystem18/1(Wheels_Rotation_Angle[rad]) -> Gain31/1
  Subsystem17/1(Wheels_Rotation_Angle[rad]) -> Gain27/1
  Subsystem16/1(Wheels_Rotation_Angle[rad]) -> Gain23/1
  Subsystem15/1(Wheels_Rotation_Angle[rad]) -> Gain19/1
  Subsystem14/1(Wheels_Rotation_Angle[rad]) -> Gain15/1
  Subsystem13/1(Wheels_Rotation_Angle[rad]) -> Gain11/1
  Subsystem12/1(Wheels_Rotation_Angle[rad]) -> Gain7/1
  Subsystem11/1(Wheels_Rotation_Angle[rad]) -> Gain3/1
  Bus Selector9/4 -> Gain38/1  "<Heading_fellow10[deg]>"
  Bus Selector9/2 -> Gain37/1  "<y_fellow10[m]>"
  Bus Selector9/1 -> Gain36/1  "<x_fellow10[m]>"
  Bus Selector9/3 -> Subsystem10/1(In1)  "<z_fellow10[m]>"
  Bus Selector8/4 -> Gain34/1  "<Heading_fellow9[deg]>"
  Bus Selector8/2 -> Gain33/1  "<y_fellow9[m]>"
  Bus Selector8/1 -> Gain32/1  "<x_fellow9[m]>"
  Bus Selector8/3 -> Subsystem9/1(In1)  "<z_fellow9[m]>"
  Bus Selector7/4 -> Gain30/1  "<Heading_fellow8[deg]>"
  Bus Selector7/2 -> Gain29/1  "<y_fellow8[m]>"
  Bus Selector7/1 -> Gain28/1  "<x_fellow8[m]>"
  Bus Selector7/3 -> Subsystem8/1(In1)  "<z_fellow8[m]>"
  Bus Selector6/4 -> Gain26/1  "<Heading_fellow7[deg]>"
  Bus Selector6/2 -> Gain25/1  "<y_fellow7[m]>"
  Bus Selector6/1 -> Gain24/1  "<x_fellow7[m]>"
  Bus Selector6/3 -> Subsystem7/1(In1)  "<z_fellow7[m]>"
  Bus Selector5/4 -> Gain22/1  "<Heading_fellow6[deg]>"
  Bus Selector5/2 -> Gain21/1  "<y_fellow6[m]>"
  Bus Selector5/1 -> Gain20/1  "<x_fellow6[m]>"
  Bus Selector5/3 -> Subsystem6/1(In1)  "<z_fellow6[m]>"
  Bus Selector4/4 -> Gain18/1  "<Heading_fellow5[deg]>"
  Bus Selector4/2 -> Gain17/1  "<y_fellow5[m]>"
  Bus Selector4/1 -> Gain16/1  "<x_fellow5[m]>"
  Bus Selector4/3 -> Subsystem5/1(In1)  "<z_fellow5[m]>"
  Bus Selector3/4 -> Gain14/1  "<Heading_fellow4[deg]>"
  Bus Selector3/2 -> Gain13/1  "<y_fellow4[m]>"
  Bus Selector3/1 -> Gain12/1  "<x_fellow4[m]>"
  Bus Selector3/3 -> Subsystem4/1(In1)  "<z_fellow4[m]>"
  Bus Selector2/4 -> Gain10/1  "<Heading_fellow3[deg]>"
  Bus Selector2/2 -> Gain9/1  "<y_fellow3[m]>"
  Bus Selector2/1 -> Gain8/1  "<x_fellow3[m]>"
  Bus Selector2/3 -> Subsystem2/1(In1)  "<z_fellow3[m]>"
  Bus Selector1/4 -> Gain6/1  "<Heading_fellow2[deg]>"
  Bus Selector1/2 -> Gain5/1  "<y_fellow2[m]>"
  Bus Selector1/1 -> Gain4/1  "<x_fellow2[m]>"
  Bus Selector1/3 -> Subsystem1/1(In1)  "<z_fellow2[m]>"
  FeedBack/1 -> Bus Selector/1, Bus Selector1/1, Bus Selector2/1, Bus Selector3/1, Bus Selector4/1, Bus Selector5/1, Bus Selector6/1, Bus Selector7/1, Bus Selector8/1, Bus Selector9/1
  Subsystem4/1(Out1) -> Gain59/1
  Subsystem2/1(Out1) -> Gain58/1
  Subsystem1/1(Out1) -> Gain57/1
  Ground25/1 -> Gain55/1
  Ground24/1 -> Gain54/1
  Ground23/1 -> Gain53/1
  Ground22/1 -> Gain52/1
  Ground21/1 -> Gain51/1
  Ground20/1 -> Gain50/1
  Ground19/1 -> Gain49/1
  Ground18/1 -> Gain48/1
  Ground17/1 -> Gain45/1
  Ground16/1 -> Gain47/1
  Ground15/1 -> Gain46/1
  Ground14/1 -> Gain44/1
  Ground13/1 -> Gain43/1
  Ground12/1 -> Gain42/1
  Ground11/1 -> Gain41/1
  Ground10/1 -> Gain40/1
  Bus Selector/4 -> Gain2/1  "<Heading_fellow1[deg]>"
  Bus Selector/3 -> Subsystem/1(In1)  "<z_fellow1[m]>"
  Bus Selector/2 -> Gain1/1  "<y_fellow1[m]>"
  Bus Selector/1 -> Gain/1  "<x_fellow1[m]>"
  Subsystem/1(Out1) -> Gain56/1
  Constant13/1 -> Gain69/1
  Constant12/1 -> Gain68/1
  Constant11/1 -> Gain67/1
  Constant10/1 -> Gain66/1
  Subsystem10/1(Out1) -> Gain65/1
  Subsystem9/1(Out1) -> Gain64/1
  Subsystem8/1(Out1) -> Gain63/1
  Subsystem7/1(Out1) -> Gain62/1
  Subsystem6/1(Out1) -> Gain61/1
  Subsystem5/1(Out1) -> Gain60/1
  Gain55/1 -> Bus Creator13/5  "Vehicle_14_Wheels_Rotation_Angle[deg]"
  Gain54/1 -> Bus Creator13/4  "Vehicle_14_Gear_Angle[deg]"
  Gain69/1 -> Bus Creator13/3  "Vehicle_14_z[m]"
  Gain53/1 -> Bus Creator13/2  "Vehicle_14_y[m]"
  Gain52/1 -> Bus Creator13/1  "Vehicle_14_x[m]"
  Gain51/1 -> Bus Creator12/5  "Vehicle_13_Wheels_Rotation_Angle[deg]"
  Gain50/1 -> Bus Creator12/4  "Vehicle_13_Gear_Angle[deg]"
  Gain68/1 -> Bus Creator12/3  "Vehicle_13_z[m]"
  Gain49/1 -> Bus Creator12/2  "Vehicle_13_y[m]"
  Gain48/1 -> Bus Creator12/1  "Vehicle_13_x[m]"
  Gain45/1 -> Bus Creator11/5  "Vehicle_12_Wheels_Rotation_Angle[deg]"
  Gain47/1 -> Bus Creator11/4  "Vehicle_12_Gear_Angle[deg]"
  Gain67/1 -> Bus Creator11/3  "Vehicle_12_z[m]"
  Gain46/1 -> Bus Creator11/2  "Vehicle_12_y[m]"
  Gain44/1 -> Bus Creator11/1  "Vehicle_12_x[m]"
  Gain43/1 -> Bus Creator10/5  "Vehicle_11_Wheels_Rotation_Angle[deg]"
  Gain42/1 -> Bus Creator10/4  "Vehicle_11_Gear_Angle[deg]"
  Gain66/1 -> Bus Creator10/3  "Vehicle_11_z[m]"
  Gain41/1 -> Bus Creator10/2  "Vehicle_11_y[m]"
  Gain40/1 -> Bus Creator10/1  "Vehicle_11_x[m]"
  Gain39/1 -> Bus Creator9/5  "Vehicle_10_Wheels_Rotation_Angle[deg]"
  Gain38/1 -> Bus Creator9/4  "Vehicle_10_Gear_Angle[deg]"
  Gain65/1 -> Bus Creator9/3  "Vehicle_10_z[m]"
  Gain37/1 -> Bus Creator9/2  "Vehicle_10_y[m]"
  Gain36/1 -> Bus Creator9/1  "Vehicle_10_x[m]"
  Gain35/1 -> Bus Creator8/5  "Vehicle_9_Wheels_Rotation_Angle[deg]"
  Gain34/1 -> Bus Creator8/4  "Vehicle_9_Gear_Angle[deg]"
  Gain64/1 -> Bus Creator8/3  "Vehicle_9_z[m]"
  Gain33/1 -> Bus Creator8/2  "Vehicle_9_y[m]"
  Gain32/1 -> Bus Creator8/1  "Vehicle_9_x[m]"
  Gain31/1 -> Bus Creator7/5  "Vehicle_8_Wheels_Rotation_Angle[deg]"
  Gain30/1 -> Bus Creator7/4  "Vehicle_8_Gear_Angle[deg]"
  Gain63/1 -> Bus Creator7/3  "Vehicle_8_z[m]"
  Gain29/1 -> Bus Creator7/2  "Vehicle_8_y[m]"
  Gain28/1 -> Bus Creator7/1  "Vehicle_8_x[m]"
  Gain27/1 -> Bus Creator6/5  "Vehicle_7_Wheels_Rotation_Angle[deg]"
  Gain26/1 -> Bus Creator6/4  "Vehicle_7_Gear_Angle[deg]"
  Gain62/1 -> Bus Creator6/3  "Vehicle_7_z[m]"
  Gain25/1 -> Bus Creator6/2  "Vehicle_7_y[m]"
  Gain24/1 -> Bus Creator6/1  "Vehicle_7_x[m]"
  Gain23/1 -> Bus Creator5/5  "Vehicle_6_Wheels_Rotation_Angle[deg]"
  Gain22/1 -> Bus Creator5/4  "Vehicle_6_Gear_Angle[deg]"
  Gain61/1 -> Bus Creator5/3  "Vehicle_6_z[m]"
  Gain21/1 -> Bus Creator5/2  "Vehicle_6_y[m]"
  Gain20/1 -> Bus Creator5/1  "Vehicle_6_x[m]"
  Gain19/1 -> Bus Creator4/5  "Vehicle_5_Wheels_Rotation_Angle[deg]"
  Gain18/1 -> Bus Creator4/4  "Vehicle_5_Gear_Angle[deg]"
  Gain60/1 -> Bus Creator4/3  "Vehicle_5_z[m]"
  Gain17/1 -> Bus Creator4/2  "Vehicle_5_y[m]"
  Gain16/1 -> Bus Creator4/1  "Vehicle_5_x[m]"
  Gain15/1 -> Bus Creator3/5  "Vehicle_4_Wheels_Rotation_Angle[deg]"
  Gain14/1 -> Bus Creator3/4  "Vehicle_4_Gear_Angle[deg]"
  Gain59/1 -> Bus Creator3/3  "Vehicle_4_z[m]"
  Gain13/1 -> Bus Creator3/2  "Vehicle_4_y[m]"
  Gain12/1 -> Bus Creator3/1  "Vehicle_4_x[m]"
  Gain11/1 -> Bus Creator2/5  "Vehicle_3_Wheels_Rotation_Angle[deg]"
  Gain10/1 -> Bus Creator2/4  "Vehicle_3_Gear_Angle[deg]"
  Gain58/1 -> Bus Creator2/3  "Vehicle_3_z[m]"
  Gain9/1 -> Bus Creator2/2  "Vehicle_3_y[m]"
  Gain8/1 -> Bus Creator2/1  "Vehicle_3_x[m]"
  Gain7/1 -> Bus Creator1/5  "Vehicle_2_Wheels_Rotation_Angle[deg]"
  Gain6/1 -> Bus Creator1/4  "Vehicle_2_Gear_Angle[deg]"
  Gain57/1 -> Bus Creator1/3  "Vehicle_2_z[m]"
  Gain5/1 -> Bus Creator1/2  "Vehicle_2_y[m]"
  Gain4/1 -> Bus Creator1/1  "Vehicle_2_x[m]"
  Gain3/1 -> Bus Creator/5  "Vehicle_1_Wheels_Rotation_Angle[deg]"
  Gain2/1 -> Bus Creator/4  "Vehicle_1_Gear_Angle[deg]"
  Gain56/1 -> Bus Creator/3  "Vehicle_1_z[m]"
  Gain1/1 -> Bus Creator/2  "Vehicle_1_y[m]"
  Gain/1 -> Bus Creator/1  "Vehicle_1_x[m]"
  Bus Creator13/1 -> Vehicle_14_Vector/1  "Vehicle_14_Vector"
  Bus Creator12/1 -> Vehicle_13_Vector/1  "Vehicle_13_Vector"
  Bus Creator11/1 -> Vehicle_12_Vector/1  "Vehicle_12_Vector"
  Bus Creator10/1 -> Vehicle_11_Vector/1  "Vehicle_11_Vector"
  Bus Creator9/1 -> Vehicle_10_Vector/1  "Vehicle_10_Vector"
  Bus Creator8/1 -> Vehicle_9_Vector/1  "Vehicle_9_Vector"
  Bus Creator7/1 -> Vehicle_8_Vector/1  "Vehicle_8_Vector"
  Bus Creator6/1 -> Vehicle_7_Vector/1  "Vehicle_7_Vector"
  Bus Creator5/1 -> Vehicle_6_Vector/1  "Vehicle_6_Vector"
  Bus Creator4/1 -> Vehicle_5_Vector/1  "Vehicle_5_Vector"
  Bus Creator3/1 -> Vehicle_4_Vector3/1  "Vehicle_4_Vector3"
  Bus Creator2/1 -> Vehicle_3_Vector/1  "Vehicle_3_Vector"
  Bus Creator1/1 -> Vehicle_2_Vector/1  "Vehicle_2_Vector"
  Bus Creator/1 -> Vehicle_1_Vector/1  "Vehicle_1_Vector"

== system PC_Simulator_Lib/Comunication_with_visualisation_normal_mode_new_Version/Subsystem3 ==
  In1 : Inport
  Add : Sum
  Constant : Constant  Value=1000
  Gain1 : Gain  Gain=60/(2*pi)
  Out1 : Outport
  wires:
  Constant/1 -> Add/2
  Gain1/1 -> Add/1
  Add/1 -> Out1/1
  In1/1 -> Gain1/1

== system PC_Simulator_Lib/Comunication_with_visualisation_normal_mode_new_Version/Subsystem4 ==
  In1 : Inport
  Gain : Gain  Gain=1/radiusWheel
  Integrator : Integrator
  Out1 : Outport
  wires:
  Gain/1 -> Integrator/1
  In1/1 -> Gain/1
  Integrator/1 -> Out1/1

== system PC_Simulator_Lib/Comunication_with_visualisation_normal_mode_new_Version/Subsystem5 ==
  In1 : Inport
  Add : Sum
  Bus Selector3 : BusSelector  OutputSignals=Vehicle_Dynamics.Wheel_Steering_Angle_Left[rad],Vehicle_Dynamics.Wheel_Steering_Angle_Right[rad]
  Gain : Gain  Gain=-0.5
  Gain1 : Gain  Gain=180/pi
  Out1 : Outport
  wires:
  Gain1/1 -> Out1/1
  Gain/1 -> Gain1/1
  Add/1 -> Gain/1
  Bus Selector3/2 -> Add/2  "<Wheel_Steering_Angle_Right[rad]>"
  Bus Selector3/1 -> Add/1  "<Wheel_Steering_Angle_Left[rad]>"
  In1/1 -> Bus Selector3/1

== system PC_Simulator_Lib/Comunication_with_visualisation_normal_mode_new_Version/Subsystem6 ==
  In1 : Inport
  Add : Sum  Inputs=++++
  Bus Selector : BusSelector  OutputSignals=ADAS.ADAS_Systems_States.ACC_State,ADAS.ADAS_Systems_States.Pilotiertes_Fahren_State,ADAS.ADAS_Systems_States.Emergency_Brake_State,ADAS.ADAS_Systems_States.Emergency_Steering_State
  Gain : Gain  Gain=4
  Gain1 : Gain  Gain=18
  Gain2 : Gain  Gain=9
  Gain3 : Gain  Gain=20
  Memory{1..4} (4 alike) : Memory
  Out1 : Outport
  wires:
  Bus Selector/1 -> Memory1/1  "<ACC_State>"
  Bus Selector/2 -> Memory2/1  "<Pilotiertes_Fahren_State>"
  Memory1/1 -> Gain/1
  Memory2/1 -> Gain1/1
  Add/1 -> Out1/1
  Gain/1 -> Add/1
  Gain1/1 -> Add/2
  Bus Selector/3 -> Memory3/1  "<Emergency_Brake_State>"
  Memory3/1 -> Gain2/1
  Gain2/1 -> Add/3
  Gain3/1 -> Add/4
  Memory4/1 -> Gain3/1
  Bus Selector/4 -> Memory4/1  "<Emergency_Steering_State>"
  In1/1 -> Bus Selector/1

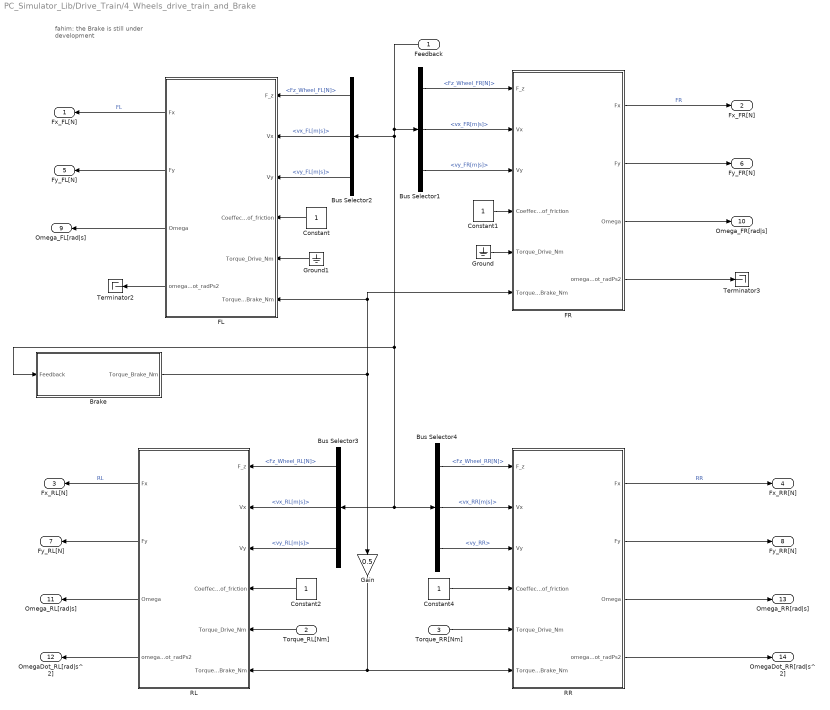
== system PC_Simulator_Lib/Drive_Train/4_Wheels_drive_train_and_Brake ==
  note: fahim:
      | the Brake is still under development
  Feedback : Inport
  Torque_RL[Nm] : Inport  Port=2
  Torque_RR[Nm] : Inport  Port=3
  Brake : Subsystem
  Bus Selector1 : BusSelector  OutputSignals=Vehicle_Dynamics.Fz_Wheel.Fz_Wheel_FR[N],Vehicle_Dynamics.Velocity_Wheels[m|s].v_FR[m|s].vx_FR[m|s],Vehicle_Dynamics.Velocity_Wheels[m|s].v_FR[m|s].vy_FR[m|s]
  Bus Selector2 : BusSelector  OutputSignals=Vehicle_Dynamics.Fz_Wheel.Fz_Wheel_FL[N],Vehicle_Dynamics.Velocity_Wheels[m|s].v_FL[m|s].vx_FL[m|s],Vehicle_Dynamics.Velocity_Wheels[m|s].v_FL[m|s].vy_FL[m|s]
  Bus Selector3 : BusSelector  OutputSignals=Vehicle_Dynamics.Fz_Wheel.Fz_Wheel_RL[N],Vehicle_Dynamics.Velocity_Wheels[m|s].v_RL[m|s].vx_RL[m|s],Vehicle_Dynamics.Velocity_Wheels[m|s].v_RL[m|s].vy_RL[m|s]
  Bus Selector4 : BusSelector  OutputSignals=Vehicle_Dynamics.Fz_Wheel.Fz_Wheel_RR[N],Vehicle_Dynamics.Velocity_Wheels[m|s].v_RR[m|s].vx_RR[m|s],Vehicle_Dynamics.Velocity_Wheels[m|s].v_RR[m|s].vy_RR
  Constant{,1..2,4} (4 alike) : Constant
  FL : Subsystem
  FR : Subsystem
  Gain : Gain  Gain=0.5
  Ground : Ground
  Ground1 : Ground
  RL : Subsystem
  RR : Subsystem
  Terminator2 : Terminator
  Terminator3 : Terminator
  Fx_FL[N] : Outport
  Fx_FR[N] : Outport  Port=2
  Fx_RL[N] : Outport  Port=3
  Fx_RR[N] : Outport  Port=4
  Fy_FL[N] : Outport  Port=5
  Fy_FR[N] : Outport  Port=6
  Fy_RL[N] : Outport  Port=7
  Fy_RR[N] : Outport  Port=8
  Omega_FL[rad|s] : Outport  Port=9
  Omega_FR[rad|s] : Outport  Port=10
  Omega_RL[rad|s] : Outport  Port=11
  OmegaDot_RL[rad|s^2] : Outport  Port=12
  Omega_RR[rad|s] : Outport  Port=13
  OmegaDot_RR[rad|s^2] : Outport  Port=14
  wires:
  RL/2(Fy) -> Fy_RL[N]/1
  FL/2(Fy) -> Fy_FL[N]/1
  FR/2(Fy) -> Fy_FR[N]/1
  RR/1(Fx) -> Fx_RR[N]/1  "RR"
  RL/1(Fx) -> Fx_RL[N]/1  "RL"
  RR/3(Omega) -> Omega_RR[rad|s]/1
  RL/3(Omega) -> Omega_RL[rad|s]/1
  FR/1(Fx) -> Fx_FR[N]/1  "FR"
  FL/1(Fx) -> Fx_FL[N]/1  "FL"
  Feedback/1 -> Bus Selector3/1, Bus Selector4/1, Brake/1(Feedback), Bus Selector2/1, Bus Selector1/1
  Bus Selector2/1 -> FL/1(F_z)  "<Fz_Wheel_FL[N]>"
  Bus Selector2/2 -> FL/2(Vx)  "<vx_FL[m|s]>"
  Bus Selector2/3 -> FL/3(Vy)  "<vy_FL[m|s]>"
  Constant/1 -> FL/4(Coeffecient_of_friction)
  Constant1/1 -> FR/4(Coeffecient_of_friction)
  Bus Selector1/1 -> FR/1(F_z)  "<Fz_Wheel_FR[N]>"
  Bus Selector1/2 -> FR/2(Vx)  "<vx_FR[m|s]>"
  Bus Selector1/3 -> FR/3(Vy)  "<vy_FR[m|s]>"
  Constant2/1 -> RL/4(Coeffecient_of_friction)
  Bus Selector3/1 -> RL/1(F_z)  "<Fz_Wheel_RL[N]>"
  Bus Selector3/2 -> RL/2(Vx)  "<vx_RL[m|s]>"
  Bus Selector3/3 -> RL/3(Vy)  "<vy_RL[m|s]>"
  Bus Selector4/1 -> RR/1(F_z)  "<Fz_Wheel_RR[N]>"
  Bus Selector4/2 -> RR/2(Vx)  "<vx_RR[m|s]>"
  Bus Selector4/3 -> RR/3(Vy)  "<vy_RR>"
  Constant4/1 -> RR/4(Coeffecient_of_friction)
  RR/2(Fy) -> Fy_RR[N]/1
  RR/4(omegaDot_radPs2) -> OmegaDot_RR[rad|s^2]/1
  RL/4(omegaDot_radPs2) -> OmegaDot_RL[rad|s^2]/1
  FR/3(Omega) -> Omega_FR[rad|s]/1
  FL/3(Omega) -> Omega_FL[rad|s]/1
  Torque_RL[Nm]/1 -> RL/5(Torque_Drive_Nm)
  Brake/1(Torque_Brake_Nm) -> Gain/1, FL/6(Torque_Brake_Nm), FR/6(Torque_Brake_Nm)
  Torque_RR[Nm]/1 -> RR/5(Torque_Drive_Nm)
  Gain/1 -> RL/6(Torque_Brake_Nm), RR/6(Torque_Brake_Nm)
  Ground/1 -> FR/5(Torque_Drive_Nm)
  Ground1/1 -> FL/5(Torque_Drive_Nm)
  FL/4(omegaDot_radPs2) -> Terminator2/1
  FR/4(omegaDot_radPs2) -> Terminator3/1

== system PC_Simulator_Lib/Drive_Train/Differential ==
  Torque_in : Inport
  rotation_1 : Inport  Port=2
  rotation_2 : Inport  Port=3
  Add : Sum
  Add1 : Sum
  Demux : Demux  Outputs=2
  Demux1 : Demux  Outputs=2
  Gain : Gain  Gain=0.5
  Gain1 : Gain  Gain=0.5
  Gain2 : Gain  Gain=0.5
  Ground : Ground
  Memory : Memory
  Subtract1 : Sum  Inputs=+-
  Terminator : Terminator
  moment_of_inertia1 : Gain  Gain=inertiaLateral
  uebersetzung : Gain  Gain=Para.DT.Differential_Gear_ratio.v
  uebersetzung1 : Gain  Gain=Para.DT.Differential_Gear_ratio.v
  uebersetzung2 : Gain  Gain=Para.DT.Differential_Gear_ratio.v
  Torque_out_1 : Outport
  Torque_out_2 : Outport  Port=2
  omega_out_gearbox_radPs : Outport  Port=3
  omegaDot_out_gearbox_radPs1 : Outport  Port=4
  wires:
  Torque_in/1 -> uebersetzung1/1
  Add/1 -> Gain/1
  Gain/1 -> uebersetzung/1
  uebersetzung/1 -> omega_out_gearbox_radPs/1
  Gain1/1 -> Torque_out_1/1, Torque_out_2/1
  rotation_1/1 -> Demux/1
  rotation_2/1 -> Demux1/1
  Demux/1 -> Add/1
  Demux1/1 -> Add/2
  Add1/1 -> Gain2/1
  Gain2/1 -> uebersetzung2/1, Memory/1
  Demux/2 -> Add1/1
  Demux1/2 -> Add1/2
  uebersetzung1/1 -> Subtract1/1
  uebersetzung2/1 -> omegaDot_out_gearbox_radPs1/1
  Subtract1/1 -> Gain1/1
  Memory/1 -> moment_of_inertia1/1
  moment_of_inertia1/1 -> Terminator/1
  Ground/1 -> Subtract1/2

== system PC_Simulator_Lib/Drive_Train/Engine ==
  Throttle : Inport
  Omega_engine_radPs : Inport  Port=2
  OmegaDot_engine_radPs2 : Inport  Port=3
  Compare To Constant : simulink/Logic and Bit Operations/Compare To Constant  relop=<=  const=omega_max  OutDataTypeStr=uint8
  Engine_Map : Lookup_n-D  NumberOfTableDimensions=1  BreakpointsForDimension1=eng_speed  BeginIndexSearchUsingPreviousIndexResult=on  Table=torque  InputSameDT=on
  Gain1 : Gain  Gain=60/(2*pi)
  Ground : Ground
  Memory : Memory
  Product : Product  Inputs=3  RndMeth=Zero
  Saturation : Saturate  UpperLimit=1  LowerLimit=0
  Subtract : Sum  Inputs=+-+
  Terminator : Terminator
  friction : Lookup_n-D  NumberOfTableDimensions=1  BreakpointsForDimension1=omega_engine  BeginIndexSearchUsingPreviousIndexResult=on  Table=Torque_lost  InputSameDT=on
  moment_of_inertia : Gain  Gain=Para.DT.Flywheel_Inertia.v*10
  Torque : Outport
  wires:
  Throttle/1 -> Saturation/1
  Saturation/1 -> Product/1
  Engine_Map/1 -> Product/2
  Omega_engine_radPs/1 -> Gain1/1
  Product/1 -> Subtract/1
  Compare To Constant/1 -> Product/3
  Gain1/1 -> Engine_Map/1, Compare To Constant/1, friction/1
  moment_of_inertia/1 -> Terminator/1
  Subtract/1 -> Torque/1
  OmegaDot_engine_radPs2/1 -> Memory/1
  Memory/1 -> moment_of_inertia/1
  friction/1 -> Subtract/3
  Ground/1 -> Subtract/2

== system PC_Simulator_Lib/Drive_Train/Gearbox ==
  velocity : Inport
  DNR : Inport  Port=2
  Torque_Engine : Inport  Port=3
  omega_out_gearbox_radPs : Inport  Port=4
  omegaDot_out_gearbox_radPs2 : Inport  Port=5
  Automatic_Gear_box_Controller : Stateflow chart  TreatAsAtomicUnit=on
  Multiport Switch : MultiPortSwitch  DataPortOrder=Zero-based contiguous  Inputs=7  zeroidx=on
  Product : Product  RndMeth=Zero
  Product1 : Product  RndMeth=Zero
  Product2 : Product  RndMeth=Zero
  Saturation : Saturate  UpperLimit=6  LowerLimit=0
  fifth_gear : Constant  Value=Para.DT.Fifth_Gear_reduction_Ratio.v
  first_gear : Constant  Value=Para.DT.First_Gear_reduction_Ratio.v
  fouth_gear : Constant  Value=Para.DT.Forth_Gear_reduction_Ratio.v
  neutral : Constant  Value=0
  neutral1 : Constant  Value=5000
  reverse : Constant  Value=Para.DT.Reverse_Gear_reduction_Ratio.v
  second_gear : Constant  Value=Para.DT.Second_Gear_reduction_Ratio.v
  third_gear : Constant  Value=Para.DT.Third_Gear_reduction_Ratio.v
  omega_engine_radPs : Outport
  Torque_out_gearbox_Nm : Outport  Port=2
  omegaDot_engine_radPs2 : Outport  Port=3
  Gearbox_Gear_Ratio : Outport  Port=4
  wires:
  DNR/1 -> Automatic_Gear_box_Controller/2(DNR)
  Saturation/1 -> Multiport Switch/1
  Multiport Switch/1 -> Product1/1, Product2/1, Product/1, Gearbox_Gear_Ratio/1
  Torque_Engine/1 -> Product/2
  Product/1 -> Torque_out_gearbox_Nm/1
  Product1/1 -> omega_engine_radPs/1
  Automatic_Gear_box_Controller/1(gear) -> Saturation/1
  neutral/1 -> Multiport Switch/2
  velocity/1 -> Automatic_Gear_box_Controller/1(velocity)
  neutral1/1 -> Automatic_Gear_box_Controller/3(omega)
  omega_out_gearbox_radPs/1 -> Product1/2
  omegaDot_out_gearbox_radPs2/1 -> Product2/2
  Product2/1 -> omegaDot_engine_radPs2/1
  first_gear/1 -> Multiport Switch/3
  second_gear/1 -> Multiport Switch/4
  third_gear/1 -> Multiport Switch/5
  fouth_gear/1 -> Multiport Switch/6
  fifth_gear/1 -> Multiport Switch/7
  reverse/1 -> Multiport Switch/8

== system PC_Simulator_Lib/Drive_Train/Output_Interface ==
  Force_tire_x_FL[N] : Inport
  Force_tire_x_FR[N] : Inport  Port=2
  Force_tire_x_RL[N] : Inport  Port=3
  Force_tire_x_RR[N] : Inport  Port=4
  Force_tire_y_FL[N] : Inport  Port=5
  Force_tire_y_FR[N] : Inport  Port=6
  Force_tire_y_RL[N] : Inport  Port=7
  Force_tire_y_RR[N] : Inport  Port=8
  Omega_FL[rad|s] : Inport  Port=9
  Omega_FR[rad|s] : Inport  Port=10
  Omega_RL[rad|s] : Inport  Port=11
  Omega_RR[rad|s] : Inport  Port=12
  Omega_Engine[rad|s] : Inport  Port=13
  Gearbox_Gear_Ratio : Inport  Port=14
  Bus Creator : BusCreator  Inputs=5
  Bus Creator1 : BusCreator
  Bus Creator2 : BusCreator
  Bus Creator3 : BusCreator
  Gain{,1..11} (12 alike) : Gain
  Drive_Train : Outport
  wires:
  Bus Creator1/1 -> Bus Creator/1  "Force_x_tire[N]"
  Bus Creator2/1 -> Bus Creator/2  "Force_y_tire[N]"
  Force_tire_x_FL[N]/1 -> Gain11/1
  Force_tire_x_FR[N]/1 -> Gain10/1
  Force_tire_x_RL[N]/1 -> Gain9/1
  Bus Creator/1 -> Drive_Train/1  "Drive_Train"
  Force_tire_x_RR[N]/1 -> Gain8/1
  Force_tire_y_FL[N]/1 -> Gain7/1
  Force_tire_y_FR[N]/1 -> Gain6/1
  Force_tire_y_RL[N]/1 -> Gain5/1
  Force_tire_y_RR[N]/1 -> Gain4/1
  Omega_FL[rad|s]/1 -> Gain/1
  Omega_FR[rad|s]/1 -> Gain1/1
  Omega_RL[rad|s]/1 -> Gain2/1
  Omega_RR[rad|s]/1 -> Gain3/1
  Bus Creator3/1 -> Bus Creator/3  "Omega_4_Wheels[rad|s]"
  Gain/1 -> Bus Creator3/1  "Omega_FL[rad|s]"
  Gain1/1 -> Bus Creator3/2  "Omega_FR[rad|s]"
  Gain2/1 -> Bus Creator3/3  "Omega_RL[rad|s]"
  Gain3/1 -> Bus Creator3/4  "Omega_RR[rad|s]"
  Gain4/1 -> Bus Creator2/4  "Force_tire_y_RR[N]"
  Gain5/1 -> Bus Creator2/3  "Force_tire_y_RL[N]"
  Gain6/1 -> Bus Creator2/2  "Force_tire_y_FR[N]"
  Gain7/1 -> Bus Creator2/1  "Force_tire_y_FL[N]"
  Gain8/1 -> Bus Creator1/4  "Force_tire_x_RR[N]"
  Gain9/1 -> Bus Creator1/3  "Force_tire_x_RL[N]"
  Gain10/1 -> Bus Creator1/2  "Force_tire_x_FR[N]"
  Gain11/1 -> Bus Creator1/1  "Force_tire_x_FL[N]"
  Omega_Engine[rad|s]/1 -> Bus Creator/4  "Omega_Engine[rad|s]"
  Gearbox_Gear_Ratio/1 -> Bus Creator/5  "Gearbox_Gear_Ratio"
